simulink model "estimator_ukf_v02"  (Simulink 7.0)
settings: Solver=FixedStepDiscrete  StartTime=0  StopTime=10  FixedStep=ts  RelTol=1e-3
undefined symbols (not defined in the file): c, Ilf, Irf, l_fts, m, n, P0, Q, R, ROBOT, ts, W, WM, X0
libraries: simulink x5
settings Model: Creator=raje_ra  LastModifiedBy=raje_ra  ExtModeAutoUpdateStatusClock=off

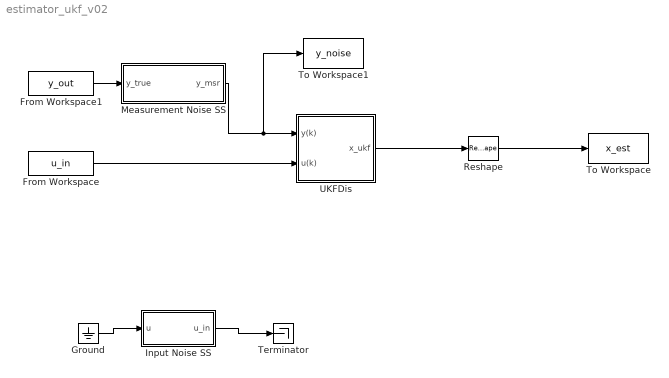
== system estimator_ukf_v02 ==
  From Workspace : FromWorkspace  VariableName=u_in  SampleTime=0
  From Workspace1 : FromWorkspace  VariableName=y_out  SampleTime=0
  Ground : Ground
  Input Noise SS : Subsystem
  Measurement Noise SS : Subsystem
  Reshape : Reshape
  Terminator : Terminator
  To Workspace : ToWorkspace  VariableName=x_est  SampleTime=-1  SaveFormat=Structure With Time
  To Workspace1 : ToWorkspace  VariableName=y_noise  SampleTime=-1  SaveFormat=Structure With Time
  UKFDis : Subsystem
  wires:
  UKFDis/1(x_ukf) -> Reshape/1
  From Workspace1/1 -> Measurement Noise SS/1(y_true)
  From Workspace/1 -> UKFDis/2(u(k))
  Reshape/1 -> To Workspace/1
  Measurement Noise SS/1(y_msr) -> UKFDis/1(y(k)), To Workspace1/1
  Ground/1 -> Input Noise SS/1(u)
  Input Noise SS/1(u_in) -> Terminator/1

== system estimator_ukf_v02/Input Noise SS ==
  note: Noise with Sandard Deviation 1e-1 is added to inputs
  u : Inport  OutDataType=sfix(16)  OutScaling=2^0
  Band-Limited White Noise1 : simulink/Sources/Band-Limited White Noise  SystemSampleTime=-1  Cov=[1e-5]  Ts=ts  seed=[23341]
  Sum : Sum  Inputs=|++  OutDataType=sfix(16)  OutScaling=2^0
  u_in : Outport
  wires:
  Band-Limited White Noise1/1 -> Sum/2
  Sum/1 -> u_in/1
  u/1 -> Sum/1

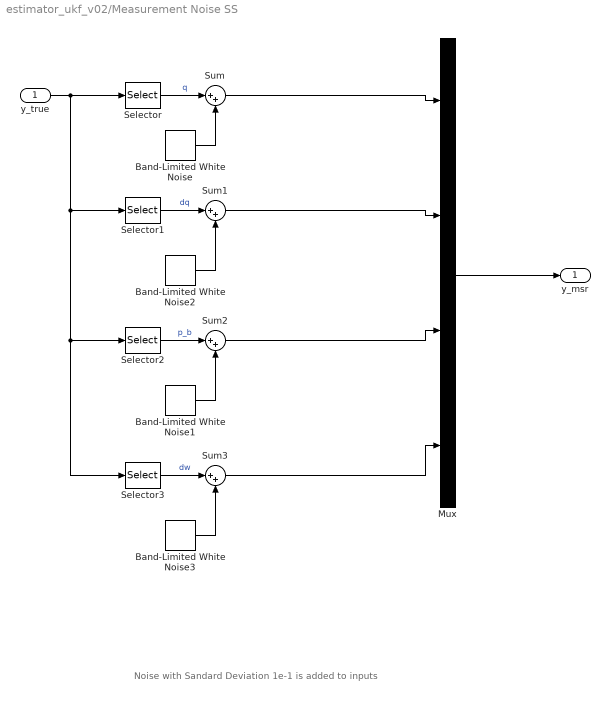
== system estimator_ukf_v02/Measurement Noise SS ==
  note: Noise with Sandard Deviation 1e-1 is added to inputs
  y_true : Inport  OutDataType=sfix(16)  OutScaling=2^0
  Band-Limited White Noise : simulink/Sources/Band-Limited White Noise  SystemSampleTime=-1  Cov=[1e-9]  Ts=ts  seed=[23341]
  Band-Limited White Noise1 : simulink/Sources/Band-Limited White Noise  SystemSampleTime=-1  Cov=[1e-5]  Ts=ts  seed=[23341]
  Band-Limited White Noise2 : simulink/Sources/Band-Limited White Noise  SystemSampleTime=-1  Cov=[1e-7]  Ts=ts  seed=[23341]
  Band-Limited White Noise3 : simulink/Sources/Band-Limited White Noise  SystemSampleTime=-1  Cov=[1e-7]  Ts=ts  seed=[23341]
  Mux : Mux
  Selector : Selector  InputPortWidth=m  IndexOptions=Index vector (dialog)  Indices=[1:25]  OutputSizes=1
  Selector1 : Selector  InputPortWidth=m  IndexOptions=Index vector (dialog)  Indices=[26:50]  OutputSizes=1
  Selector2 : Selector  InputPortWidth=m  IndexOptions=Index vector (dialog)  Indices=[51:53]  OutputSizes=1
  Selector3 : Selector  InputPortWidth=m  IndexOptions=Index vector (dialog)  Indices=[54:56]  OutputSizes=1
  Sum{,1..3} (4 alike) : Sum  Inputs=|++  OutDataType=sfix(16)  OutScaling=2^0
  y_msr : Outport
  wires:
  Mux/1 -> y_msr/1
  Sum3/1 -> Mux/4
  Sum2/1 -> Mux/3
  Sum1/1 -> Mux/2
  Sum/1 -> Mux/1
  Selector3/1 -> Sum3/1  "dw"
  Band-Limited White Noise3/1 -> Sum3/2
  Selector2/1 -> Sum2/1  "p_b"
  Band-Limited White Noise1/1 -> Sum2/2
  Band-Limited White Noise2/1 -> Sum1/2
  Selector1/1 -> Sum1/1  "dq"
  Selector/1 -> Sum/1  "q"
  y_true/1 -> Selector3/1, Selector2/1, Selector1/1, Selector/1
  Band-Limited White Noise/1 -> Sum/2

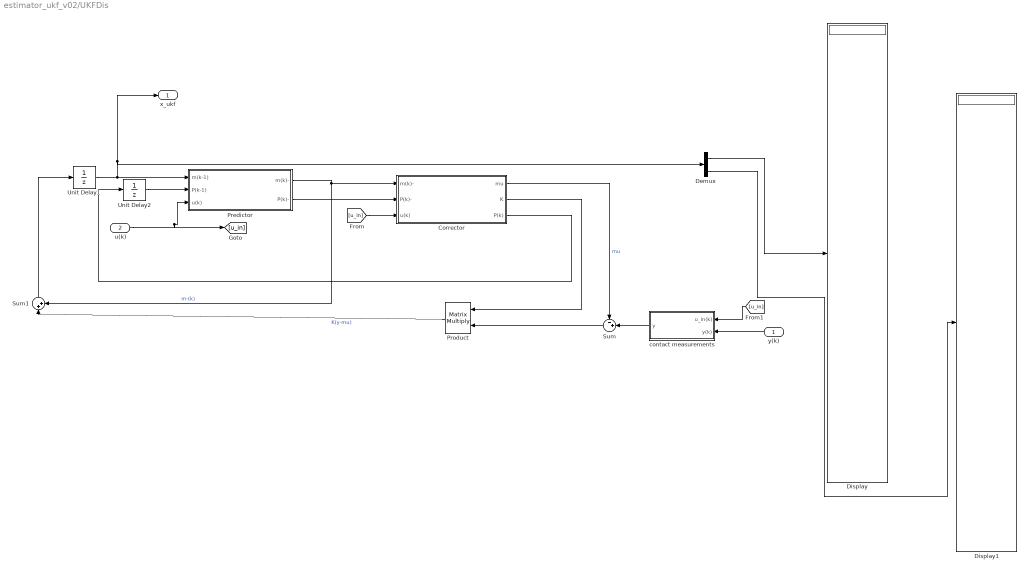
== system estimator_ukf_v02/UKFDis ==
  y(k) : Inport  Orientation=left
  u(k) : Inport  Port=2
  Corrector : Subsystem
  Demux : Demux  Outputs=2
  Display : Display
  Display1 : Display
  Predictor : Subsystem
  Product : Product  Orientation=left  Multiplication=Matrix(*)  OutDataType=sfix(16)  OutScaling=2^0  RndMeth=Zero
  Sum : Sum  Orientation=left  Inputs=-+|  OutDataType=sfix(16)  OutScaling=2^0
  Sum1 : Sum  Orientation=up  Inputs=|++  OutDataType=sfix(16)  OutScaling=2^0
  Unit Delay1 : UnitDelay  X0=X0  SampleTime=-1
  Unit Delay2 : UnitDelay  X0=P0  SampleTime=-1
  contact measurements : Subsystem  Orientation=left
  x_ukf : Outport  OutDataType=sfix(16)  OutScaling=2^0
  wires:
  Sum1/1 -> Unit Delay1/1
  Unit Delay1/1 -> Predictor/1(m(k-1)), x_ukf/1, Demux/1
  Predictor/1(m(k)-) -> Sum1/2, Corrector/1(m(k)-)  "m-(k)"
  Predictor/2(P(k)-) -> Corrector/2(P(k)-)
  Corrector/1(mu) -> Sum/1  "mu"
  Corrector/2(K) -> Product/1
  Sum/1 -> Product/2
  Product/1 -> Sum1/1  "K(y-mu)"
  Unit Delay2/1 -> Predictor/2(P(k-1))
  Corrector/3(P(k)) -> Unit Delay2/1
  u(k)/1 -> Predictor/3(u(k)), [u_in]
  [u_in] -> Corrector/3(u(k))
  contact measurements/1(y) -> Sum/2
  [u_in] -> contact measurements/1(u_in(k))
  y(k)/1 -> contact measurements/2(y(k))
  Demux/1 -> Display/1
  Demux/2 -> Display1/1

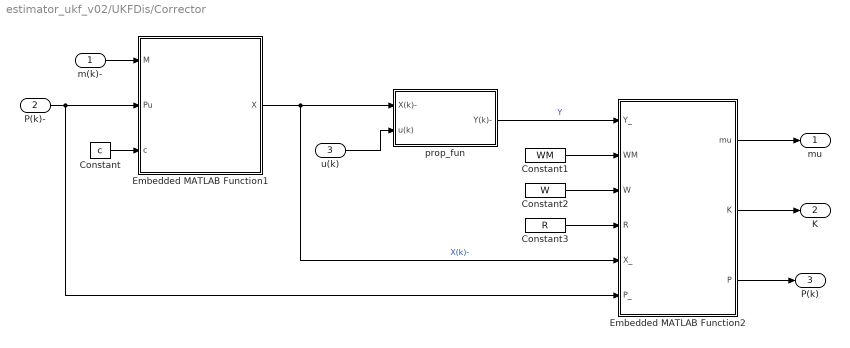
== system estimator_ukf_v02/UKFDis/Corrector ==
  m(k)- : Inport
  P(k)- : Inport  Port=2
  u(k) : Inport  Port=3
  Constant : Constant  Value=c  OutDataType=sfix(16)  OutScaling=2^0
  Constant1 : Constant  Value=WM  VectorParams1D=off  OutDataType=sfix(16)  OutScaling=2^0
  Constant2 : Constant  Value=W  VectorParams1D=off  OutDataType=sfix(16)  OutScaling=2^0
  Constant3 : Constant  Value=R  VectorParams1D=off  OutDataType=sfix(16)  OutScaling=2^0
  Embedded MATLAB Function1 : Stateflow chart
  Embedded MATLAB Function2 : Stateflow chart
  prop_fun : Subsystem
  mu : Outport
  K : Outport  Port=2
  P(k) : Outport  Port=3
  wires:
  u(k)/1 -> prop_fun/2(u(k))
  m(k)-/1 -> Embedded MATLAB Function1/1(M)
  P(k)-/1 -> Embedded MATLAB Function1/2(Pu), Embedded MATLAB Function2/6(P_)
  Constant/1 -> Embedded MATLAB Function1/3(c)
  Embedded MATLAB Function1/1(X) -> prop_fun/1(X(k)-), Embedded MATLAB Function2/5(X_)  "X(k)-"
  prop_fun/1(Y(k)-) -> Embedded MATLAB Function2/1(Y_)  "Y"
  Constant1/1 -> Embedded MATLAB Function2/2(WM)
  Constant2/1 -> Embedded MATLAB Function2/3(W)
  Constant3/1 -> Embedded MATLAB Function2/4(R)
  Embedded MATLAB Function2/1(mu) -> mu/1
  Embedded MATLAB Function2/2(K) -> K/1
  Embedded MATLAB Function2/3(P) -> P(k)/1

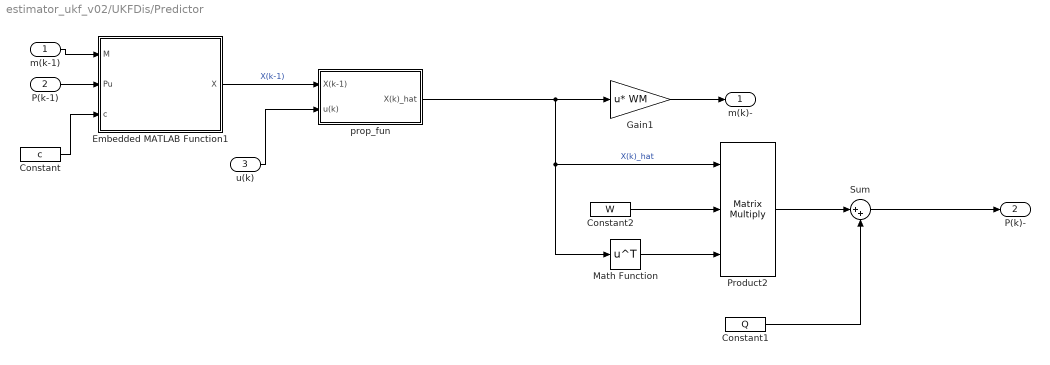
== system estimator_ukf_v02/UKFDis/Predictor ==
  m(k-1) : Inport
  P(k-1) : Inport  Port=2
  u(k) : Inport  Port=3
  Constant : Constant  Value=c  OutDataType=sfix(16)  OutScaling=2^0
  Constant1 : Constant  Value=Q  OutDataType=sfix(16)  OutScaling=2^0
  Constant2 : Constant  Value=W  OutDataType=sfix(16)  OutScaling=2^0
  Embedded MATLAB Function1 : Stateflow chart
  Gain1 : Gain  Gain=WM  Multiplication=Matrix(u*K)  ParameterDataType=sfix(16)  ParameterScaling=2^0  OutDataType=sfix(16)  OutScaling=2^0
  Math Function : Math  Operator=transpose  OutDataType=sfix(16)  OutScaling=2^0  SaturateOnIntegerOverflow=on
  Product2 : Product  Inputs=3  Multiplication=Matrix(*)  OutDataType=sfix(16)  OutScaling=2^0  RndMeth=Zero
  Sum : Sum  Inputs=|++  OutDataType=sfix(16)  OutScaling=2^0
  prop_fun : Subsystem
  m(k)- : Outport
  P(k)- : Outport  Port=2
  wires:
  u(k)/1 -> prop_fun/2(u(k))
  Embedded MATLAB Function1/1(X) -> prop_fun/1(X(k-1))  "X(k-1)"
  Product2/1 -> Sum/1
  Constant1/1 -> Sum/2
  Sum/1 -> P(k)-/1
  Constant/1 -> Embedded MATLAB Function1/3(c)
  m(k-1)/1 -> Embedded MATLAB Function1/1(M)
  P(k-1)/1 -> Embedded MATLAB Function1/2(Pu)
  Gain1/1 -> m(k)-/1
  prop_fun/1(X(k)_hat) -> Gain1/1, Math Function/1, Product2/1  "X(k)_hat"
  Constant2/1 -> Product2/2
  Math Function/1 -> Product2/3

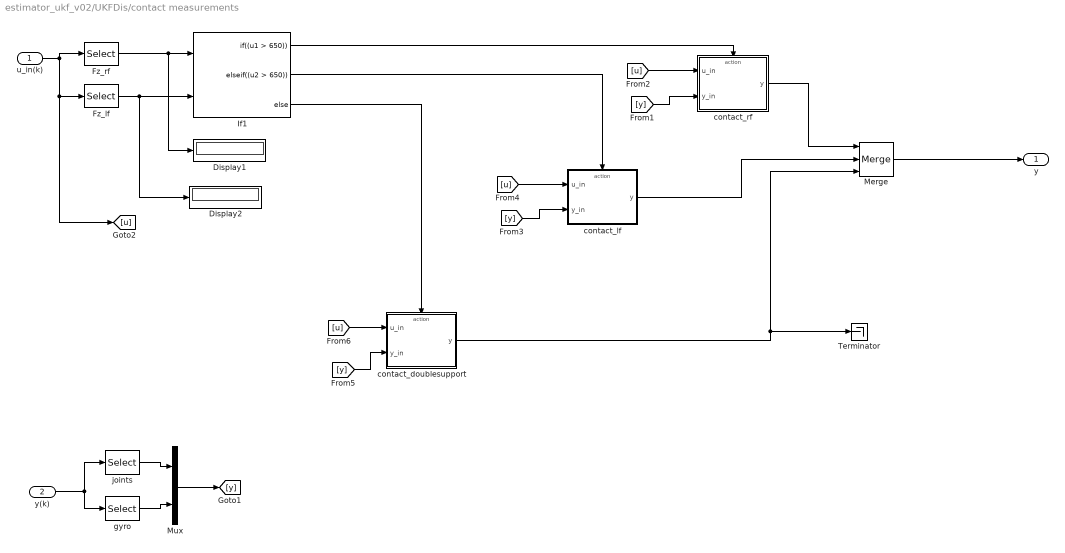
== system estimator_ukf_v02/UKFDis/contact measurements ==
  u_in(k) : Inport
  y(k) : Inport  Port=2
  Display1 : Display
  Display2 : Display
  Fz_lf : Selector  InputPortWidth=37  IndexOptions=Index vector (dialog)  Indices=3  OutputSizes=1
  Fz_rf : Selector  InputPortWidth=37  IndexOptions=Index vector (dialog)  Indices=3  OutputSizes=1
  If1 : If  NumInputs=2  IfExpression=(u1 > 650)  ElseIfExpressions=(u2 > 650)
  Merge : Merge  Inputs=3
  Mux : Mux  Inputs=2
  Terminator : Terminator
  contact_doublesupport : Subsystem
  contact_lf : Subsystem
  contact_rf : Subsystem
  gyro : Selector  InputPortWidth=56  IndexOptions=Index vector (dialog)  Indices=[51:56]  OutputSizes=1
  joints : Selector  InputPortWidth=56  IndexOptions=Index vector (dialog)  Indices=1:50  OutputSizes=1
  y : Outport
  wires:
  Mux/1 -> [y]
  gyro/1 -> Mux/2
  joints/1 -> Mux/1
  contact_doublesupport/1(y) -> Merge/3, Terminator/1
  Merge/1 -> y/1
  contact_lf/1(y) -> Merge/2
  contact_rf/1(y) -> Merge/1
  If1/3 -> contact_doublesupport/Action
  If1/2 -> contact_lf/Action
  [y] -> contact_doublesupport/2(y_in)
  [u] -> contact_doublesupport/1(u_in)
  [y] -> contact_lf/2(y_in)
  [u] -> contact_lf/1(u_in)
  [y] -> contact_rf/2(y_in)
  [u] -> contact_rf/1(u_in)
  If1/1 -> contact_rf/Action
  u_in(k)/1 -> [u], Fz_lf/1, Fz_rf/1
  Fz_lf/1 -> Display2/1, If1/2
  Fz_rf/1 -> Display1/1, If1/1
  y(k)/1 -> gyro/1, joints/1

== system estimator_ukf_v02/UKFDis/Corrector/prop_fun ==
  X(k)- : Inport
  u(k) : Inport  Port=2
  F(X) : Subsystem  TreatAsAtomicUnit=on
  Y(k)- : Outport
  wires:
  u(k)/1 -> F(X)/2(u(k))
  X(k)-/1 -> F(X)/1(X(k)-)
  F(X)/1(Y(k)-) -> Y(k)-/1

== system estimator_ukf_v02/UKFDis/Predictor/prop_fun ==
  note: 1)Forward Euler Integration: x(k) = x(k-1) ts*f(x(k-1))
  X(k-1) : Inport
  u(k) : Inport  Port=2
  F(X) : Subsystem  TreatAsAtomicUnit=on
  Gain3 : Gain  Gain=ts  ParameterDataType=sfix(16)  ParameterScaling=2^0  OutDataType=sfix(16)  OutScaling=2^0
  Sum1 : Sum  Inputs=|++  OutDataType=sfix(16)  OutScaling=2^0
  X(k)_hat : Outport
  wires:
  u(k)/1 -> F(X)/2(u(k))
  Sum1/1 -> X(k)_hat/1
  X(k-1)/1 -> Sum1/2, F(X)/1(X(k-1))
  F(X)/1(F(X)) -> Gain3/1
  Gain3/1 -> Sum1/1

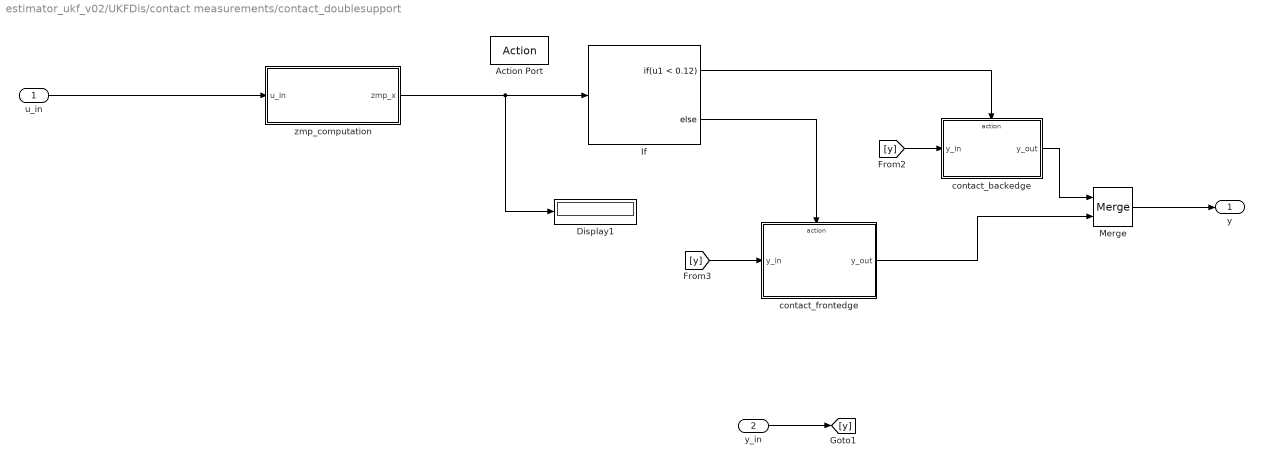
== system estimator_ukf_v02/UKFDis/contact measurements/contact_doublesupport ==
  u_in : Inport
  y_in : Inport  Port=2
  Action Port : ActionPort  ActionType=else
  Display1 : Display
  If : If  IfExpression=u1 < 0.12
  Merge : Merge
  contact_backedge : Subsystem  TreatAsAtomicUnit=on
  contact_frontedge : Subsystem  TreatAsAtomicUnit=on
  zmp_computation : Subsystem
  y : Outport
  wires:
  u_in/1 -> zmp_computation/1(u_in)
  zmp_computation/1(zmp_x) -> Display1/1, If/1
  y_in/1 -> [y]
  Merge/1 -> y/1
  contact_frontedge/1(y_out) -> Merge/2
  contact_backedge/1(y_out) -> Merge/1
  [y] -> contact_frontedge/1(y_in)
  [y] -> contact_backedge/1(y_in)
  If/2 -> contact_frontedge/Action
  If/1 -> contact_backedge/Action

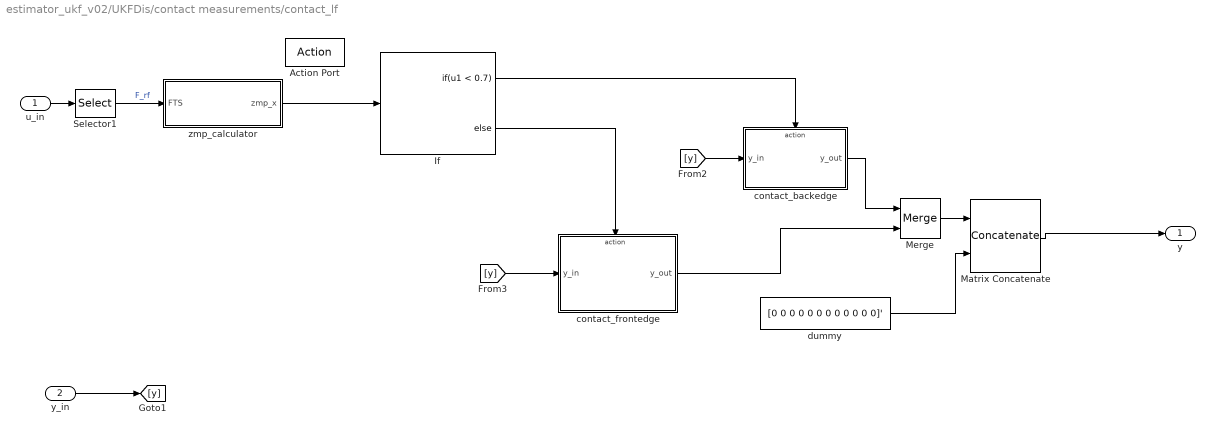
== system estimator_ukf_v02/UKFDis/contact measurements/contact_lf ==
  u_in : Inport
  y_in : Inport  Port=2
  Action Port : ActionPort  ActionType=elseif
  If : If  IfExpression=u1 < 0.7
  Matrix Concatenate : Concatenate  Mode=Multidimensional array
  Merge : Merge
  Selector1 : Selector  InputPortWidth=37  IndexOptions=Index vector (dialog)  Indices=7:12  OutputSizes=1
  contact_backedge : Subsystem  TreatAsAtomicUnit=on
  contact_frontedge : Subsystem  TreatAsAtomicUnit=on
  dummy : Constant  Value=[0 0 0 0 0 0 0 0 0 0 0 0]'  VectorParams1D=off  OutDataType=sfix(16)  OutScaling=2^0
  zmp_calculator : Subsystem
  y : Outport
  wires:
  Matrix Concatenate/1 -> y/1
  dummy/1 -> Matrix Concatenate/2
  Merge/1 -> Matrix Concatenate/1
  If/1 -> contact_backedge/Action
  If/2 -> contact_frontedge/Action
  [y] -> contact_backedge/1(y_in)
  [y] -> contact_frontedge/1(y_in)
  contact_backedge/1(y_out) -> Merge/1
  contact_frontedge/1(y_out) -> Merge/2
  zmp_calculator/1(zmp_x) -> If/1
  Selector1/1 -> zmp_calculator/1(FTS)  "F_rf"
  u_in/1 -> Selector1/1
  y_in/1 -> [y]

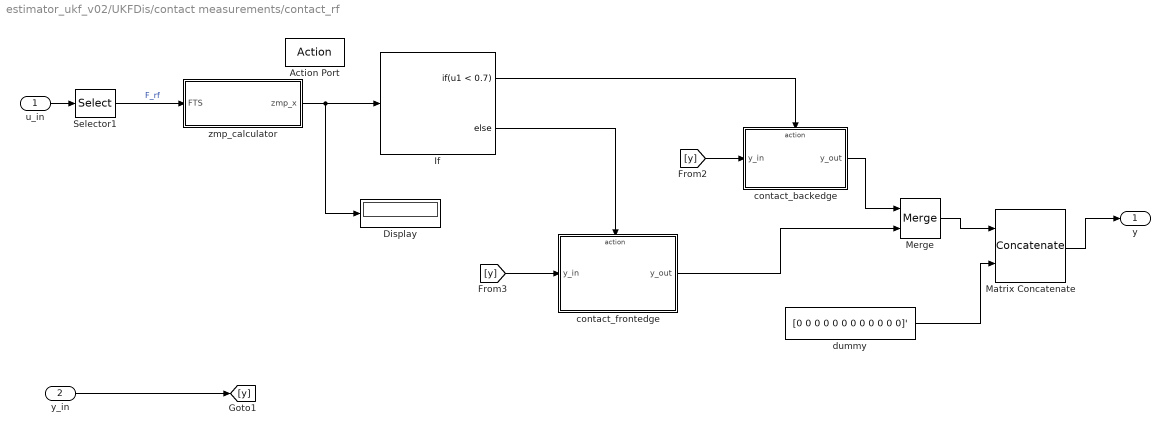
== system estimator_ukf_v02/UKFDis/contact measurements/contact_rf ==
  u_in : Inport
  y_in : Inport  Port=2
  Action Port : ActionPort  ActionType=then
  Display : Display
  If : If  IfExpression=u1 < 0.7
  Matrix Concatenate : Concatenate  Mode=Multidimensional array
  Merge : Merge
  Selector1 : Selector  InputPortWidth=37  IndexOptions=Index vector (dialog)  Indices=1:6  OutputSizes=1
  contact_backedge : Subsystem  TreatAsAtomicUnit=on
  contact_frontedge : Subsystem  TreatAsAtomicUnit=on
  dummy : Constant  Value=[0 0 0 0 0 0 0 0 0 0 0 0]'  VectorParams1D=off  OutDataType=sfix(16)  OutScaling=2^0
  zmp_calculator : Subsystem
  y : Outport
  wires:
  Matrix Concatenate/1 -> y/1
  Merge/1 -> Matrix Concatenate/1
  dummy/1 -> Matrix Concatenate/2
  y_in/1 -> [y]
  u_in/1 -> Selector1/1
  Selector1/1 -> zmp_calculator/1(FTS)  "F_rf"
  zmp_calculator/1(zmp_x) -> Display/1, If/1
  contact_frontedge/1(y_out) -> Merge/2
  contact_backedge/1(y_out) -> Merge/1
  [y] -> contact_frontedge/1(y_in)
  [y] -> contact_backedge/1(y_in)
  If/2 -> contact_frontedge/Action
  If/1 -> contact_backedge/Action

== system estimator_ukf_v02/UKFDis/Corrector/prop_fun/F(X) ==
  X(k)- : Inport  OutDataType=sfix(16)  OutScaling=2^0
  u(k) : Inport  Port=2  OutDataType=sfix(16)  OutScaling=2^0
  Assignment : Assignment  NumberOfDimensions=2  IndexOptions=Assign all,Index vector (port)  Indices=1,1  OutputSizes=2,2
  Constant : Constant  Value=zeros(m+24,2*n+1)  VectorParams1D=off  OutDataType=sfix(16)  OutScaling=2^0  SampleTime=-1
  Display : Display
  For Iterator : ForIterator  ResetStates=reset  IterationLimit=2*n +1  IterationVariableDataType=double
  Reshape : Reshape  OutputDimensionality=Column vector (2-D)
  Selector : Selector  NumberOfDimensions=2  IndexOptions=Select all,Index vector (port)  Indices=[1 3],1  OutputSizes=1,1
  dyn_model : Subsystem
  Y(k)- : Outport  OutDataType=sfix(16)  OutScaling=2^0
  wires:
  u(k)/1 -> dyn_model/2(u_in(k))
  Constant/1 -> Assignment/1
  Assignment/1 -> Y(k)-/1
  dyn_model/1(y(k)) -> Reshape/1
  Selector/1 -> dyn_model/1(x(k-1))
  For Iterator/1 -> Display/1, Assignment/3, Selector/2
  X(k)-/1 -> Selector/1
  Reshape/1 -> Assignment/2

== system estimator_ukf_v02/UKFDis/Predictor/prop_fun/F(X) ==
  X(k-1) : Inport  OutDataType=sfix(16)  OutScaling=2^0
  u(k) : Inport  Port=2  OutDataType=sfix(16)  OutScaling=2^0
  Assignment : Assignment  NumberOfDimensions=2  IndexOptions=Assign all,Index vector (port)  Indices=1,1  OutputSizes=2,2
  For Iterator : ForIterator  ResetStates=reset  IterationLimit=2*n +1  IterationVariableDataType=double
  Reshape : Reshape  OutputDimensionality=Column vector (2-D)
  Selector : Selector  NumberOfDimensions=2  IndexOptions=Select all,Index vector (port)  Indices=[1 3],1  OutputSizes=1,1
  dyn_model : Subsystem
  F(X) : Outport  OutDataType=sfix(16)  OutScaling=2^0
  wires:
  Assignment/1 -> F(X)/1
  dyn_model/1(f(x(k-1))) -> Reshape/1
  Selector/1 -> dyn_model/1(x(k-1))
  For Iterator/1 -> Selector/2, Assignment/3
  X(k-1)/1 -> Assignment/1, Selector/1
  u(k)/1 -> dyn_model/2(u_in(k))
  Reshape/1 -> Assignment/2

== system estimator_ukf_v02/UKFDis/contact measurements/contact_doublesupport/contact_backedge ==
  y_in : Inport  OutDataType=sfix(16)  OutScaling=2^0
  Action Port : ActionPort  ActionType=then
  Matrix Concatenate : Concatenate  NumInputs=4  Mode=Multidimensional array
  V_feet : Constant  Value=[0 0 0 0 0 0 0 0 0 0 0 0]'  VectorParams1D=off  OutDataType=sfix(16)  OutScaling=2^0
  lf_contact_CD : Constant  Value="[-0.059999942250943   0.065450013201346  -0.000099999469068  -0.059999926220207   0.160450013201344  -0.000099995026751]'"  VectorParams1D=off  OutDataType=sfix(16)  OutScaling=2^0
  rf_contact_CD : Constant  Value="[-0.059999991262275  -0.160449976611997  -0.000099795625568  -0.059999972932080  -0.065449976612284  -0.000099562918613]'"  VectorParams1D=off  OutDataType=sfix(16)  OutScaling=2^0
  y_out : Outport  OutDataType=sfix(16)  OutScaling=2^0
  wires:
  V_feet/1 -> Matrix Concatenate/4
  lf_contact_CD/1 -> Matrix Concatenate/3
  rf_contact_CD/1 -> Matrix Concatenate/2
  Matrix Concatenate/1 -> y_out/1
  y_in/1 -> Matrix Concatenate/1

== system estimator_ukf_v02/UKFDis/contact measurements/contact_doublesupport/contact_frontedge ==
  y_in : Inport  OutDataType=sfix(16)  OutScaling=2^0
  Action Port : ActionPort  ActionType=else
  Matrix Concatenate : Concatenate  NumInputs=4  Mode=Multidimensional array
  V_feet : Constant  Value=[0 0 0 0 0 0 0 0 0 0 0 0]'  VectorParams1D=off  OutDataType=sfix(16)  OutScaling=2^0
  lf_contact_AB : Constant  Value="[0.130000073779718   0.160449981139864  -0.000099828958185   0.130000057748982   0.065449981139865  -0.000099833400502]'"  VectorParams1D=off  OutDataType=sfix(16)  OutScaling=2^0
  rf_contact_AB : Constant  Value="[0.130000027067808  -0.065450013272176  -0.000099766533171   0.130000008737612  -0.160450013271890  -0.000099999240125]'"  VectorParams1D=off  OutDataType=sfix(16)  OutScaling=2^0
  y_out : Outport  OutDataType=sfix(16)  OutScaling=2^0
  wires:
  V_feet/1 -> Matrix Concatenate/4
  lf_contact_AB/1 -> Matrix Concatenate/3
  rf_contact_AB/1 -> Matrix Concatenate/2
  Matrix Concatenate/1 -> y_out/1
  y_in/1 -> Matrix Concatenate/1

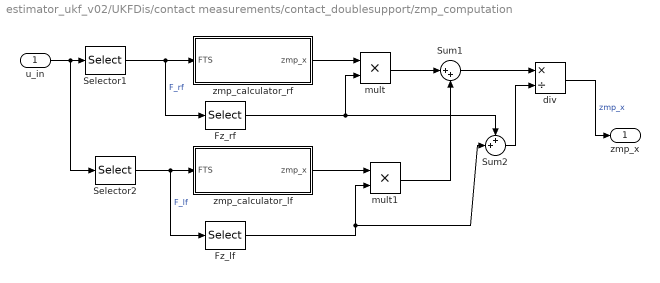
== system estimator_ukf_v02/UKFDis/contact measurements/contact_doublesupport/zmp_computation ==
  u_in : Inport
  Fz_lf : Selector  InputPortWidth=6  IndexOptions=Index vector (dialog)  Indices=3  OutputSizes=1
  Fz_rf : Selector  InputPortWidth=6  IndexOptions=Index vector (dialog)  Indices=3  OutputSizes=1
  Selector1 : Selector  InputPortWidth=37  IndexOptions=Index vector (dialog)  Indices=1:6  OutputSizes=1
  Selector2 : Selector  InputPortWidth=37  IndexOptions=Index vector (dialog)  Indices=7:12  OutputSizes=1
  Sum1 : Sum  Inputs=|++  OutDataType=sfix(16)  OutScaling=2^0
  Sum2 : Sum  Inputs=++|  OutDataType=sfix(16)  OutScaling=2^0
  div : Product  Inputs=*/  OutDataType=sfix(16)  OutScaling=2^-10
  mult : Product  Inputs=**  OutDataType=sfix(16)  OutScaling=2^-10
  mult1 : Product  Inputs=**  OutDataType=sfix(16)  OutScaling=2^-10
  zmp_calculator_lf : Subsystem
  zmp_calculator_rf : Subsystem
  zmp_x : Outport
  wires:
  div/1 -> zmp_x/1  "zmp_x"
  Sum2/1 -> div/2
  Sum1/1 -> div/1
  mult1/1 -> Sum1/2
  zmp_calculator_lf/1(zmp_x) -> mult1/1
  mult/1 -> Sum1/1
  zmp_calculator_rf/1(zmp_x) -> mult/1
  Fz_rf/1 -> Sum2/1, mult/2
  Fz_lf/1 -> Sum2/2, mult1/2
  Selector2/1 -> Fz_lf/1, zmp_calculator_lf/1(FTS)  "F_lf"
  u_in/1 -> Selector2/1, Selector1/1
  Selector1/1 -> Fz_rf/1, zmp_calculator_rf/1(FTS)  "F_rf"

== system estimator_ukf_v02/UKFDis/contact measurements/contact_lf/contact_backedge ==
  y_in : Inport  OutDataType=sfix(16)  OutScaling=2^0
  Action Port : ActionPort  ActionType=then
  Matrix Concatenate : Concatenate  NumInputs=3  Mode=Multidimensional array
  V_lf : Constant  Value=[0 0 0 0 0 0]'  VectorParams1D=off  OutDataType=sfix(16)  OutScaling=2^0
  lf_contact_CD : Constant  Value="[-0.059999942250943   0.065450013201346  -0.000099999469068  -0.059999926220207   0.160450013201344  -0.000099995026751]'"  VectorParams1D=off  OutDataType=sfix(16)  OutScaling=2^0
  y_out : Outport  OutDataType=sfix(16)  OutScaling=2^0
  wires:
  lf_contact_CD/1 -> Matrix Concatenate/2
  y_in/1 -> Matrix Concatenate/1
  Matrix Concatenate/1 -> y_out/1
  V_lf/1 -> Matrix Concatenate/3

== system estimator_ukf_v02/UKFDis/contact measurements/contact_lf/contact_frontedge ==
  y_in : Inport  OutDataType=sfix(16)  OutScaling=2^0
  Action Port : ActionPort  ActionType=else
  Matrix Concatenate : Concatenate  NumInputs=3  Mode=Multidimensional array
  V_lf : Constant  Value=[0 0 0 0 0 0]'  VectorParams1D=off  OutDataType=sfix(16)  OutScaling=2^0
  lf_contact_AB : Constant  Value="[0.130000073779718   0.160449981139864  -0.000099828958185   0.130000057748982   0.065449981139865  -0.000099833400502]'"  VectorParams1D=off  OutDataType=sfix(16)  OutScaling=2^0
  y_out : Outport  OutDataType=sfix(16)  OutScaling=2^0
  wires:
  V_lf/1 -> Matrix Concatenate/3
  lf_contact_AB/1 -> Matrix Concatenate/2
  y_in/1 -> Matrix Concatenate/1
  Matrix Concatenate/1 -> y_out/1

== system estimator_ukf_v02/UKFDis/contact measurements/contact_lf/zmp_calculator ==
  FTS : Inport
  Demux : Demux  Outputs=6
  Divide : Product  Inputs=*/  OutDataType=sfix(16)  OutScaling=2^-10
  Divide1 : Product  Inputs=/*  OutDataType=sfix(16)  OutScaling=2^-10
  Gain : Gain  Gain=l_fts  ParameterDataType=sfix(16)  ParameterScaling=2^0  OutDataType=sfix(16)  OutScaling=2^0
  Gain1 : Gain  Gain=l_fts  ParameterDataType=sfix(16)  ParameterScaling=2^0  OutDataType=sfix(16)  OutScaling=2^0
  Sum : Sum  Inputs=|--  OutDataType=sfix(16)  OutScaling=2^0
  Sum1 : Sum  Inputs=+-|  OutDataType=sfix(16)  OutScaling=2^0
  Terminator : Terminator
  Terminator1 : Terminator
  zmp_x : Outport
  wires:
  Demux/1 -> Gain/1
  Gain/1 -> Sum/1
  Demux/5 -> Sum/2
  Sum/1 -> Divide/1
  Demux/3 -> Divide/2, Divide1/1
  Demux/2 -> Gain1/1
  Gain1/1 -> Sum1/2
  Demux/4 -> Sum1/1
  Sum1/1 -> Divide1/2
  Demux/6 -> Terminator/1
  Divide1/1 -> Terminator1/1  "zmp_y"
  Divide/1 -> zmp_x/1  "zmp_x"
  FTS/1 -> Demux/1

== system estimator_ukf_v02/UKFDis/contact measurements/contact_rf/contact_backedge ==
  y_in : Inport  OutDataType=sfix(16)  OutScaling=2^0
  Action Port : ActionPort  ActionType=then
  Matrix Concatenate : Concatenate  NumInputs=3  Mode=Multidimensional array
  V_rf : Constant  Value=[0 0 0 0 0 0]'  VectorParams1D=off  OutDataType=sfix(16)  OutScaling=2^0
  rf_contact_CD : Constant  Value="[-0.059999991262275  -0.160449976611997  -0.000099795625568  -0.059999972932080  -0.065449976612284  -0.000099562918613]'"  VectorParams1D=off  OutDataType=sfix(16)  OutScaling=2^0
  y_out : Outport  OutDataType=sfix(16)  OutScaling=2^0
  wires:
  V_rf/1 -> Matrix Concatenate/3
  rf_contact_CD/1 -> Matrix Concatenate/2
  Matrix Concatenate/1 -> y_out/1
  y_in/1 -> Matrix Concatenate/1

== system estimator_ukf_v02/UKFDis/contact measurements/contact_rf/contact_frontedge ==
  y_in : Inport  OutDataType=sfix(16)  OutScaling=2^0
  Action Port : ActionPort  ActionType=else
  Matrix Concatenate : Concatenate  NumInputs=3  Mode=Multidimensional array
  V_rf : Constant  Value=[0 0 0 0 0 0]'  VectorParams1D=off  OutDataType=sfix(16)  OutScaling=2^0
  rf_contact_AB : Constant  Value="[0.130000027067808  -0.065450013272176  -0.000099766533171   0.130000008737612  -0.160450013271890  -0.000099999240125]'"  VectorParams1D=off  OutDataType=sfix(16)  OutScaling=2^0
  y_out : Outport  OutDataType=sfix(16)  OutScaling=2^0
  wires:
  V_rf/1 -> Matrix Concatenate/3
  rf_contact_AB/1 -> Matrix Concatenate/2
  Matrix Concatenate/1 -> y_out/1
  y_in/1 -> Matrix Concatenate/1

== system estimator_ukf_v02/UKFDis/contact measurements/contact_rf/zmp_calculator ==
  FTS : Inport
  Demux : Demux  Outputs=6
  Divide : Product  Inputs=*/  OutDataType=sfix(16)  OutScaling=2^-10
  Divide1 : Product  Inputs=/*  OutDataType=sfix(16)  OutScaling=2^-10
  Gain : Gain  Gain=l_fts  ParameterDataType=sfix(16)  ParameterScaling=2^0  OutDataType=sfix(16)  OutScaling=2^0
  Gain1 : Gain  Gain=l_fts  ParameterDataType=sfix(16)  ParameterScaling=2^0  OutDataType=sfix(16)  OutScaling=2^0
  Sum : Sum  Inputs=|--  OutDataType=sfix(16)  OutScaling=2^0
  Sum1 : Sum  Inputs=+-|  OutDataType=sfix(16)  OutScaling=2^0
  Terminator : Terminator
  Terminator1 : Terminator
  zmp_x : Outport
  wires:
  FTS/1 -> Demux/1
  Divide/1 -> zmp_x/1  "zmp_x"
  Divide1/1 -> Terminator1/1  "zmp_y"
  Demux/6 -> Terminator/1
  Sum1/1 -> Divide1/2
  Demux/4 -> Sum1/1
  Gain1/1 -> Sum1/2
  Demux/2 -> Gain1/1
  Demux/3 -> Divide1/1, Divide/2
  Sum/1 -> Divide/1
  Demux/5 -> Sum/2
  Gain/1 -> Sum/1
  Demux/1 -> Gain/1

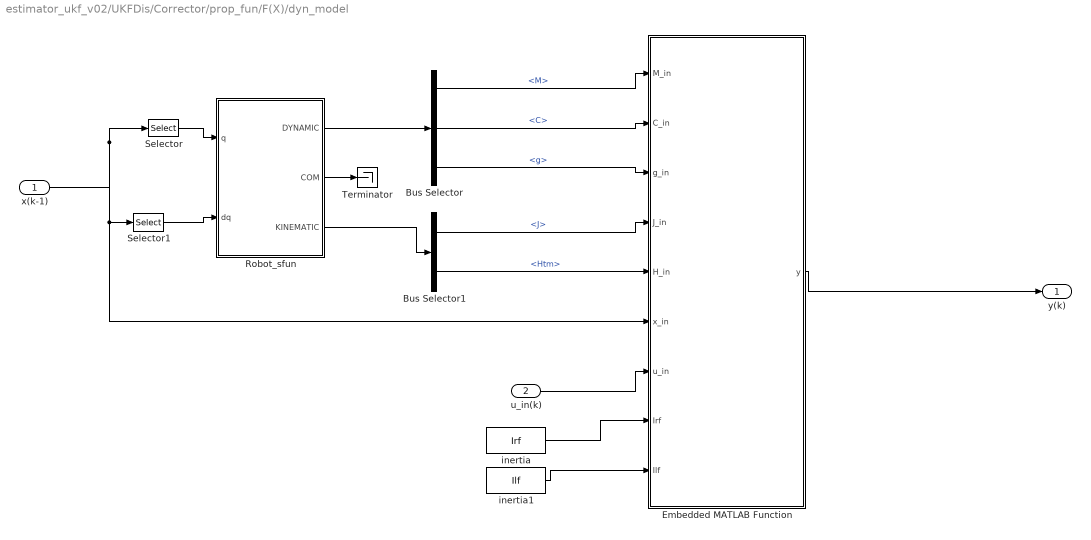
== system estimator_ukf_v02/UKFDis/Corrector/prop_fun/F(X)/dyn_model ==
  x(k-1) : Inport
  u_in(k) : Inport  Port=2
  Bus Selector : BusSelector  OutputSignals=M,C,g
  Bus Selector1 : BusSelector  OutputSignals=J,Htm
  Embedded MATLAB Function : Stateflow chart
  Robot_sfun : Subsystem
  Selector : Selector  InputPortWidth=62  IndexOptions=Index vector (dialog)  Indices=[1:31]  OutputSizes=1
  Selector1 : Selector  InputPortWidth=62  IndexOptions=Index vector (dialog)  Indices=[32:62]  OutputSizes=1
  Terminator : Terminator
  inertia : Constant  Value=Irf  VectorParams1D=off  OutDataType=sfix(16)  OutScaling=2^0
  inertia1 : Constant  Value=Ilf  VectorParams1D=off  OutDataType=sfix(16)  OutScaling=2^0
  y(k) : Outport
  wires:
  Embedded MATLAB Function/1(y) -> y(k)/1
  x(k-1)/1 -> Selector1/1, Embedded MATLAB Function/6(x_in), Selector/1
  Robot_sfun/1(DYNAMIC) -> Bus Selector/1
  Robot_sfun/3(KINEMATIC) -> Bus Selector1/1
  Selector/1 -> Robot_sfun/1(q)
  Selector1/1 -> Robot_sfun/2(dq)
  Robot_sfun/2(COM) -> Terminator/1
  Bus Selector/1 -> Embedded MATLAB Function/1(M_in)  "<M>"
  Bus Selector/2 -> Embedded MATLAB Function/2(C_in)  "<C>"
  Bus Selector/3 -> Embedded MATLAB Function/3(g_in)  "<g>"
  Bus Selector1/1 -> Embedded MATLAB Function/4(J_in)  "<J>"
  Bus Selector1/2 -> Embedded MATLAB Function/5(H_in)  "<Htm>"
  u_in(k)/1 -> Embedded MATLAB Function/7(u_in)
  inertia/1 -> Embedded MATLAB Function/8(Irf)
  inertia1/1 -> Embedded MATLAB Function/9(Ilf)

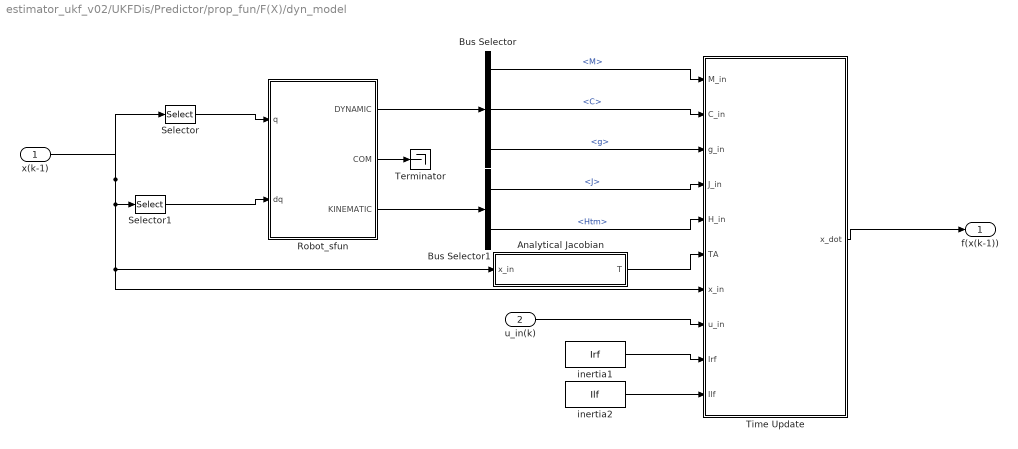
== system estimator_ukf_v02/UKFDis/Predictor/prop_fun/F(X)/dyn_model ==
  x(k-1) : Inport
  u_in(k) : Inport  Port=2
  Analytical Jacobian : Stateflow chart
  Bus Selector : BusSelector  OutputSignals=M,C,g
  Bus Selector1 : BusSelector  OutputSignals=J,Htm
  Robot_sfun : Subsystem
  Selector : Selector  InputPortWidth=62  IndexOptions=Index vector (dialog)  Indices=[1:31]  OutputSizes=1
  Selector1 : Selector  InputPortWidth=62  IndexOptions=Index vector (dialog)  Indices=[32:62]  OutputSizes=1
  Terminator : Terminator
  Time Update : Stateflow chart
  inertia1 : Constant  Value=Irf  VectorParams1D=off  OutDataType=sfix(16)  OutScaling=2^0
  inertia2 : Constant  Value=Ilf  VectorParams1D=off  OutDataType=sfix(16)  OutScaling=2^0
  f(x(k-1)) : Outport
  wires:
  Robot_sfun/1(DYNAMIC) -> Bus Selector/1
  Robot_sfun/3(KINEMATIC) -> Bus Selector1/1
  x(k-1)/1 -> Selector1/1, Analytical Jacobian/1(x_in), Time Update/7(x_in), Selector/1
  Selector/1 -> Robot_sfun/1(q)
  Selector1/1 -> Robot_sfun/2(dq)
  Robot_sfun/2(COM) -> Terminator/1
  Bus Selector/1 -> Time Update/1(M_in)  "<M>"
  Bus Selector/2 -> Time Update/2(C_in)  "<C>"
  Bus Selector/3 -> Time Update/3(g_in)  "<g>"
  Bus Selector1/1 -> Time Update/4(J_in)  "<J>"
  Bus Selector1/2 -> Time Update/5(H_in)  "<Htm>"
  Analytical Jacobian/1(T) -> Time Update/6(TA)
  u_in(k)/1 -> Time Update/8(u_in)
  Time Update/1(x_dot) -> f(x(k-1))/1
  inertia1/1 -> Time Update/9(Irf)
  inertia2/1 -> Time Update/10(Ilf)

== system estimator_ukf_v02/UKFDis/contact measurements/contact_doublesupport/zmp_computation/zmp_calculator_lf ==
  FTS : Inport
  Demux : Demux  Outputs=6
  Divide : Product  Inputs=*/  OutDataType=sfix(16)  OutScaling=2^-10
  Divide1 : Product  Inputs=/*  OutDataType=sfix(16)  OutScaling=2^-10
  Gain : Gain  Gain=l_fts  ParameterDataType=sfix(16)  ParameterScaling=2^0  OutDataType=sfix(16)  OutScaling=2^0
  Gain1 : Gain  Gain=l_fts  ParameterDataType=sfix(16)  ParameterScaling=2^0  OutDataType=sfix(16)  OutScaling=2^0
  Sum : Sum  Inputs=|--  OutDataType=sfix(16)  OutScaling=2^0
  Sum1 : Sum  Inputs=+-|  OutDataType=sfix(16)  OutScaling=2^0
  Terminator : Terminator
  Terminator1 : Terminator
  zmp_x : Outport
  wires:
  Demux/1 -> Gain/1
  Gain/1 -> Sum/1
  Demux/5 -> Sum/2
  Sum/1 -> Divide/1
  Demux/3 -> Divide/2, Divide1/1
  Demux/2 -> Gain1/1
  Gain1/1 -> Sum1/2
  Demux/4 -> Sum1/1
  Sum1/1 -> Divide1/2
  Demux/6 -> Terminator/1
  Divide1/1 -> Terminator1/1  "zmp_y"
  Divide/1 -> zmp_x/1  "zmp_x"
  FTS/1 -> Demux/1

== system estimator_ukf_v02/UKFDis/contact measurements/contact_doublesupport/zmp_computation/zmp_calculator_rf ==
  FTS : Inport
  Demux : Demux  Outputs=6
  Divide : Product  Inputs=*/  OutDataType=sfix(16)  OutScaling=2^-10
  Divide1 : Product  Inputs=/*  OutDataType=sfix(16)  OutScaling=2^-10
  Gain : Gain  Gain=l_fts  ParameterDataType=sfix(16)  ParameterScaling=2^0  OutDataType=sfix(16)  OutScaling=2^0
  Gain1 : Gain  Gain=l_fts  ParameterDataType=sfix(16)  ParameterScaling=2^0  OutDataType=sfix(16)  OutScaling=2^0
  Sum : Sum  Inputs=|--  OutDataType=sfix(16)  OutScaling=2^0
  Sum1 : Sum  Inputs=+-|  OutDataType=sfix(16)  OutScaling=2^0
  Terminator : Terminator
  Terminator1 : Terminator
  zmp_x : Outport
  wires:
  FTS/1 -> Demux/1
  Divide/1 -> zmp_x/1  "zmp_x"
  Divide1/1 -> Terminator1/1  "zmp_y"
  Demux/6 -> Terminator/1
  Sum1/1 -> Divide1/2
  Demux/4 -> Sum1/1
  Gain1/1 -> Sum1/2
  Demux/2 -> Gain1/1
  Demux/3 -> Divide1/1, Divide/2
  Sum/1 -> Divide/1
  Demux/5 -> Sum/2
  Gain/1 -> Sum/1
  Demux/1 -> Gain/1

== system estimator_ukf_v02/UKFDis/Corrector/prop_fun/F(X)/dyn_model/Robot_sfun ==
  q : Inport
  dq : Inport  Port=2
  Bus Creator : BusCreator
  Bus Creator1 : BusCreator  Inputs=3
  Bus Creator2 : BusCreator  Inputs=3
  S-Function : S-Function  FunctionName=luca_dynamics_sfun  Parameters=(size(ROBOT.csi,1)/6-1), size(ROBOT.csi,2), ROBOT.parent, ROBOT.tcp, ROBOT.g0, ROBOT.csi, ROBOT.com, ROBOT.Mass
  DYNAMIC : Outport
  COM : Outport  Port=2
  KINEMATIC : Outport  Port=3
  wires:
  Bus Creator2/1 -> KINEMATIC/1
  Bus Creator1/1 -> COM/1
  Bus Creator/1 -> DYNAMIC/1
  S-Function/10 -> Bus Creator2/3  "dJ"
  S-Function/9 -> Bus Creator2/2  "J"
  S-Function/8 -> Bus Creator2/1  "Htm"
  S-Function/7 -> Bus Creator1/3  "dJ"
  S-Function/6 -> Bus Creator1/2  "J"
  S-Function/5 -> Bus Creator1/1  "x"
  S-Function/4 -> Bus Creator/4  "dM"
  S-Function/3 -> Bus Creator/3  "g"
  S-Function/2 -> Bus Creator/2  "C"
  S-Function/1 -> Bus Creator/1  "M"
  dq/1 -> S-Function/2
  q/1 -> S-Function/1

== system estimator_ukf_v02/UKFDis/Predictor/prop_fun/F(X)/dyn_model/Robot_sfun ==
  q : Inport
  dq : Inport  Port=2
  Bus Creator : BusCreator
  Bus Creator1 : BusCreator  Inputs=3
  Bus Creator2 : BusCreator  Inputs=3
  S-Function : S-Function  FunctionName=luca_dynamics_sfun  Parameters=(size(ROBOT.csi,1)/6-1), size(ROBOT.csi,2), ROBOT.parent, ROBOT.tcp, ROBOT.g0, ROBOT.csi, ROBOT.com, ROBOT.Mass
  DYNAMIC : Outport
  COM : Outport  Port=2
  KINEMATIC : Outport  Port=3
  wires:
  q/1 -> S-Function/1
  dq/1 -> S-Function/2
  S-Function/1 -> Bus Creator/1  "M"
  S-Function/2 -> Bus Creator/2  "C"
  S-Function/3 -> Bus Creator/3  "g"
  S-Function/4 -> Bus Creator/4  "dM"
  S-Function/5 -> Bus Creator1/1  "x"
  S-Function/6 -> Bus Creator1/2  "J"
  S-Function/7 -> Bus Creator1/3  "dJ"
  S-Function/8 -> Bus Creator2/1  "Htm"
  S-Function/9 -> Bus Creator2/2  "J"
  S-Function/10 -> Bus Creator2/3  "dJ"
  Bus Creator/1 -> DYNAMIC/1
  Bus Creator1/1 -> COM/1
  Bus Creator2/1 -> KINEMATIC/1

== matlab function UKFDis/Predictor/Embedded MATLAB Function1 ==
  data: M input inherited; X output inherited; Pu input inherited; c input inherited
function X = ut_sigmas(M,Pu,c)

%A = chol(Pu)';

%%{
  A = Pu;
  L  = zeros(size(A));
  def = 1;
  for i=1:size(A,1)
      for j=1:i
          s = A(i,j);
          for k=1:j-1
              s = s - L(i,k)*L(j,k);
          end
          if j < i
              if L(j,j) > eps
                  L(i,j) = s / L(j,j);
              else
                  L(i,j) = 0;
              end
          else
              if (s < -eps)
                  s = 0;
                  def = -1;
              elseif (s < eps)
                  s = 0;
                  def = min(0,def);
              end
              L(j,j) = sqrt(s);
          end
      end
  end
  A = L;
%%}
  X = [zeros(size(M)) A -A];
  X = sqrt(c)*X + repmat(M,1,size(X,2));

== matlab function UKFDis/Corrector/Embedded MATLAB Function1 ==
  data: M input inherited; X output inherited; Pu input inherited; c input inherited
function X = ut_sigmas(M,Pu,c)

%A = chol(Pu)';

%%{
  A = Pu;
  L  = zeros(size(A));
  def = 1;
  for i=1:size(A,1)
      for j=1:i
          s = A(i,j);
          for k=1:j-1
              s = s - L(i,k)*L(j,k);
          end
          if j < i
              if L(j,j) > eps
                  L(i,j) = s / L(j,j);
              else
                  L(i,j) = 0;
              end
          else
              if (s < -eps)
                  s = 0;
                  def = -1;
              elseif (s < eps)
                  s = 0;
                  def = min(0,def);
              end
              L(j,j) = sqrt(s);
          end
      end
  end
  A = L;
%%}
  X = [zeros(size(M)) A -A];
  X = sqrt(c)*X + repmat(M,1,size(X,2));

== matlab function UKFDis/Corrector/prop_fun/F(X)/dyn_model/Embedded MATLAB Function ==
  data: M_in input inherited; y output inherited; C_in input inherited; g_in input inherited; J_in input inherited; H_in input inherited; x_in input inherited; u_in input inherited; Irf input inherited; Ilf input inherited
function y = fcn(M_in,C_in,g_in,J_in,H_in,x_in,u_in,Irf,Ilf)
% This block supports the Embedded MATLAB subset.
% See the help menu for details. 

dof = 31;
ind4 = -3:0;
ind6 = -5:0;

% Dynamic parameters
M = M_in(1:dof,:);
C = C_in(1:dof,:);
grav = g_in(1:dof);

% Kinematics
% tcp = 1 - Right Foot ; 2 - Left Foot ; 3 - Right Hand ; 4 - Left Hand ;
%       5 - Floating Base

Jrf = J_in(1*6+ind6,:);
Jlf = J_in(2*6+ind6,:);

Hrf = H_in(1*4+ind4,:);


Hlf = H_in(2*4+ind4,:);

Hfb = H_in(5*4+ind4,:);
Rfb = Hfb(1:3,1:3);


Adrf = Adjoint(Hrf);
Adlf = Adjoint(Hlf);

% state - [ position ; velocity ]
% x_in  - [   1:31   ;   32:62  ]
q = x_in(1:dof);
dq = x_in(dof+(1:dof));
omega = dq(4:6);

% inputs - [FTS_RF ; FTS _LF ; TRQ_JOINT]
% u_in   - [  1:6  ;   7:12  ;  13:37   ]
Frf = u_in(1*6+ind6,:);
Flf = u_in(2*6+ind6,:);
tau = [zeros(6,1); u_in(13:37)];

% Transformation for Angular velocities to angular rates of floating base 
% on instantaneous frame of reference. x-y-z rotations.
%TA = TA_in(1*6+ind6,:);

% Gyroscopic measurements
%gyro = Rfb'*( TA(4:6,4:6) \ (Rfb*omega) ); % ~~~~~~~~~~~~~~~~~~~~~~~~Not sure weather this is correct ????????????
 gyro = omega;                                          % Should the gyroscope be necessarily rotated ???

% Inertia correction

gacc = [ 0 0 -9.81 0 0 0]';
errrf = Irf * (Adrf\gacc) ;
errlf = Ilf * (Adlf\gacc);

% Computation of accelerations
acc = M \ (-C*dq - grav + tau + Jrf'*Adrf'*Frf + Jlf'*Adlf'*Flf - Jrf'*errrf - Jlf'*errlf);
% Gravity compensation for IMU
imu_bias = [ 0.005 0 0]';
imu = acc(1:3) + Rfb'*[0 0 9.81]'+imu_bias;

%Internal sensors
jnt = [q(7:31);dq(7:31)];

% Velocity measurements for foot contact
%v_rf = Jr*v; 
%v_lf = Jl*v;
%msr_vcont = [v_rf;v_lf];

% Position of the contact points
% Contact Model:
%        y       b---------c
%        |       |      .o |
%    x_ _|       a---------d
%
% CD --> AB === Fx: 20 --> -20
% AB --> CD === Fx: -20 --> 20

contact_AB = [ 0.13 0.0475 0 1 0.13 -0.0475 0 1]';
contact_CD = [ -0.06 -0.0475 0 1 -0.06 0.0475 0 1]';

% zmp computation
zmprf_x = ( -Frf(5) -0.1189 * Frf(1) ) / Frf(3);
zmplf_x = ( -Flf(5) -0.1189 * Flf(1) ) / Flf(3);

zmp_x = (zmprf_x * Frf(3) + zmplf_x * Flf(3))/ (Frf(3)+Flf(3));

% front edge limit = 0.12
% back edge limit = -0.055
if zmp_x < 0.12
    p1 = contact_CD(1*4+ind4);
    p2 = contact_CD(2*4+ind4);
else
    p1 = contact_AB(1*4+ind4);
    p2 = contact_AB(2*4+ind4);
end

p1rf_s = Hrf * p1;
p2rf_s = Hrf * p2;

p1lf_s = Hlf * p1;
p2lf_s = Hlf * p2;

pcont = [ p1rf_s(1:3) ; p2rf_s(1:3) ; p1lf_s(1:3) ; p2lf_s(1:3) ];

vcont = [ Jrf * dq ; Jlf * dq ];
%measurement equation 
y = [ jnt ; imu ; gyro ; pcont ; vcont ];

== matlab function UKFDis/Corrector/Embedded MATLAB Function2 ==
  data: Y_ input inherited; WM input inherited; W input inherited; R input inherited; X_ input inherited; mu output inherited; P_ input inherited; K output inherited; P output inherited
function [mu,K,P] = msr_update(Y_,WM,W,R,X_,P_)

mu = Y_ * WM;

S = Y_ * W * Y_' + R;

C = X_ * W * Y_';

K = C / S;

P = P_ - K * S * K';

== matlab function UKFDis/Predictor/prop_fun/F(X)/dyn_model/Time Update ==
  data: x_dot output inherited; M_in input inherited; C_in input inherited; g_in input inherited; J_in input inherited; H_in input inherited; TA input inherited; x_in input inherited; u_in input inherited; Irf input inherited; Ilf input inherited
function x_dot= fcn(M_in,C_in,g_in,J_in,H_in,TA,x_in,u_in,Irf,Ilf)
% This block supports the Embedded MATLAB subset.
% See the help menu for details. 

dt = 1e-3;
dof = 31;
ind4 = -3:0;
ind6 = -5:0;

% Dynamic parameters
M = M_in(1:dof,:);
C = C_in(1:dof,:);
grav = g_in(1:dof);

% Kinematics
% tcp = 1 - Right Foot ; 2 - Left Foot ; 3 - Right Hand ; 4 - Left Hand ;
%       5 - Floating Base

Jrf = J_in(1*6+ind6,:);
Jlf = J_in(2*6+ind6,:);

Hrf = H_in(1*4+ind4,:);
Hlf = H_in(2*4+ind4,:);

Hfb = H_in(5*4+ind4,:);
Rfb = Hfb(1:3,1:3);

% state - [ position ; velocity ]
% x_in  - [   1:31   ;   32:62  ]
dq = x_in(dof+(1:dof));

% inputs - [FTS_RF ; FTS _LF ; TRQ_JOINT]
% u_in   - [  1:6  ;   7:12  ;  13:37   ]
Frf = u_in(1*6+ind6,:);
Flf = u_in(2*6+ind6,:);
tau = [zeros(6,1); u_in(13:37)];

% Transformation for Angular velocities to angular rates of floating base 
% on instantaneous frame of reference. x-y-z rotations.


% Transformation from body to spacial frame:
%Adfb = Adjoint(Hfb);
Adrf = Adjoint(Hrf);
Adlf = Adjoint(Hlf);

% Transformation for the velocites of floating base
% Vfb_s = (TA\Adfb)*dq(1:6); %~~~~~~~ First Attempt

vfb = Rfb * dq(1:3);
wfb = TA\(Rfb*dq(4:6));

vel = [vfb;wfb; dq(7:31)];

gacc = [ 0 0 -9.81 0 0 0]';
errrf = Irf * (Adrf\gacc) ;
errlf = Ilf * (Adlf\gacc);

% Computation of accelerations
acc = M \ (-C*dq - grav + tau + Jrf'*Adrf'*Frf + Jlf'*Adlf'*Flf - Jrf'*errrf - Jlf'*errlf);

x_dot = [vel;acc];

== matlab function UKFDis/Predictor/prop_fun/F(X)/dyn_model/Analytical Jacobian ==
  data: T output inherited; x_in input inherited
function T = fcn(x_in)
% This block supports the Embedded MATLAB subset.
% See the help menu for details. 
% state - [ position ; velocity ]
% x_in  - [   1:31   ;   32:62  ]

ox = x_in(4);
oy = x_in(5);
% Transformation for Angular velocities to angular rates of floating base 
% on instantaneous frame of reference. x-y-z rotations.
%%{
T = [1      0           sin(oy);...
     0 cos(ox) -cos(oy)*sin(ox);...
     0 sin(ox)  cos(oy)*cos(ox)];

%T_A = [eye(3,6);zeros(3),T];

%dTx = [0,0,0 ;0,-sin(ox),-cos(oy)*cos(ox);0,cos(ox),-cos(oy)*sin(ox)];
%dTy = [0,0,cos(oy);0,0,sin(oy)*sin(ox);0,0, -sin(oy)*cos(ox)];
%%}
% T = [1      0   -sin(oy);...
%      0  cos(ox)  cos(oy)*sin(ox);...
%      0 -sin(ox)  cos(oy)*cos(ox)];
%
